simulink model "gbell_mf1_2"  (Simulink 7.2)
settings: Solver=ode45  StartTime=0.0  StopTime=10.0  RelTol=1e-3
values from neighbouring files (symbols this model uses):
  fi_1_a = -0.786    [fuzzy_controller_3_trimf_params.m]    (also in fuzzy_controller_5_gbell_params.m = 0.1768; fuzzy_controller_5_trimf_optimal_params.m; fuzzy_controller_5_trimf_params.m; fuzzy_controller_7_trimf_params.m)
  fi_1_b = -0.786    [fuzzy_controller_3_trimf_params.m]    (also in fuzzy_controller_5_gbell_params.m = 3.278; fuzzy_controller_5_trimf_optimal_params.m; fuzzy_controller_5_trimf_params.m; fuzzy_controller_7_trimf_params.m)
  fi_1_c = 0    [fuzzy_controller_3_trimf_params.m]    (also in fuzzy_controller_5_gbell_params.m = -0.7664; fuzzy_controller_5_trimf_optimal_params.m = -0.1; fuzzy_controller_5_trimf_params.m = -0.393; fuzzy_controller_7_trimf_params.m = -0.523)
settings Model: Creator=Student  LastModifiedBy=Student
settings OptimizationCC: ExpressionDepthLimit=128
settings DebuggingCC: AlgebraicLoopMsg=error  UnderspecifiedInitializationDetection=Simplified  MergeDetectMultiDrivingBlocksExec=error  SolverPrmCheckMsg=none  FcnCallInpInsideContextMsg=Enable All  StateNameClashWarn=none  StrictBusMsg=ErrorLevel1
settings HardwareCC: ProdBitPerLong=64  ProdIntDivRoundTo=Zero  ProdEndianess=LittleEndian  ProdWordSize=64  ProdHWDeviceType=Intel->x86-64
settings RTWCC: Description=Create Visual C/C++ Solution File for Simulink Coder  GenerateReport=on  RetainRTWFile=on  LaunchReport=on
settings CodeAppCC: ForceParamTrailComments=on  CustomSymbolStrType=$N$R$M_T
settings GRTTargetCC: TargetFunctionLibrary=C99 (ISO)

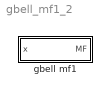
== system gbell_mf1_2 ==
  gbell mf1 : Subsystem  mask{a=fi_1_a, b=fi_1_b, c=fi_1_c}

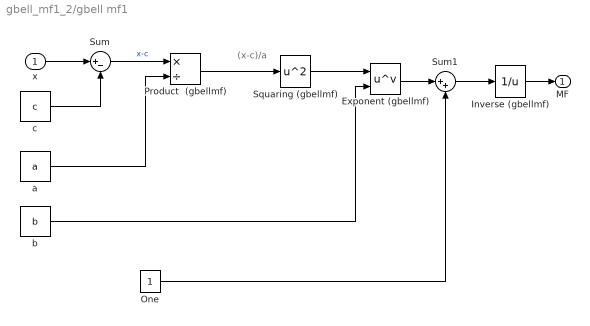
== system gbell_mf1_2/gbell mf1 ==
  note: (x-c)/a
  x : Inport
  Exponent (gbellmf) : Math  Operator=pow  SaturateOnIntegerOverflow=on
  Inverse (gbellmf) : Math  Operator=reciprocal  SaturateOnIntegerOverflow=on
  One : Constant
  Product  (gbellmf) : Product  Inputs=*/  SaturateOnIntegerOverflow=on  InputSameDT=on  OutDataTypeStr=Inherit: Same as first input
  Squaring (gbellmf) : Math  Operator=square  SaturateOnIntegerOverflow=on
  Sum : Sum  Inputs=|+-  SaturateOnIntegerOverflow=on  InputSameDT=on  OutDataTypeStr=Inherit: Same as first input
  Sum1 : Sum  Inputs=|++  SaturateOnIntegerOverflow=on  InputSameDT=on  OutDataTypeStr=Inherit: Same as first input
  a : Constant  Value=a
  b : Constant  Value=b
  c : Constant  Value=c
  MF : Outport
  wires:
  Inverse (gbellmf)/1 -> MF/1
  Sum1/1 -> Inverse (gbellmf)/1
  One/1 -> Sum1/2
  Exponent (gbellmf)/1 -> Sum1/1
  x/1 -> Sum/1
  c/1 -> Sum/2
  Sum/1 -> Product  (gbellmf)/1  "x-c"
  a/1 -> Product  (gbellmf)/2
  Product  (gbellmf)/1 -> Squaring (gbellmf)/1
  Squaring (gbellmf)/1 -> Exponent (gbellmf)/1
  b/1 -> Exponent (gbellmf)/2
